simulink model "Test_JI_dot_dot"  (R2015b)
settings: Solver=ode4  StartTime=0.0  StopTime=10  FixedStep=0.01  RelTol=1e-3
values from neighbouring files (symbols this model uses):
  D = [30,30,20,20,20,20,20,20]    [Set_Parameter.m]    (also in Set_Parameter_Single.m; Set_Parameter_line_circle.m; Set_Parameter_line_circle_DC_model_no_vision_controller.m; Set_Parameter_line_circle_no_vision_controller.m = [40,40,40,30,20,30,20,20])
  P = [60,60,50,50,30,30,20,20]    [Set_Parameter.m]    (also in Set_Parameter_Single.m; Set_Parameter_line_circle.m; Set_Parameter_line_circle_DC_model_no_vision_controller.m = [120,120,100,100,60,60,40,40]; Set_Parameter_line_circle_no_vision_controller.m = [350,100,300,150,50,100,20,20])
settings Model: Creator=User  LastModifiedBy=User

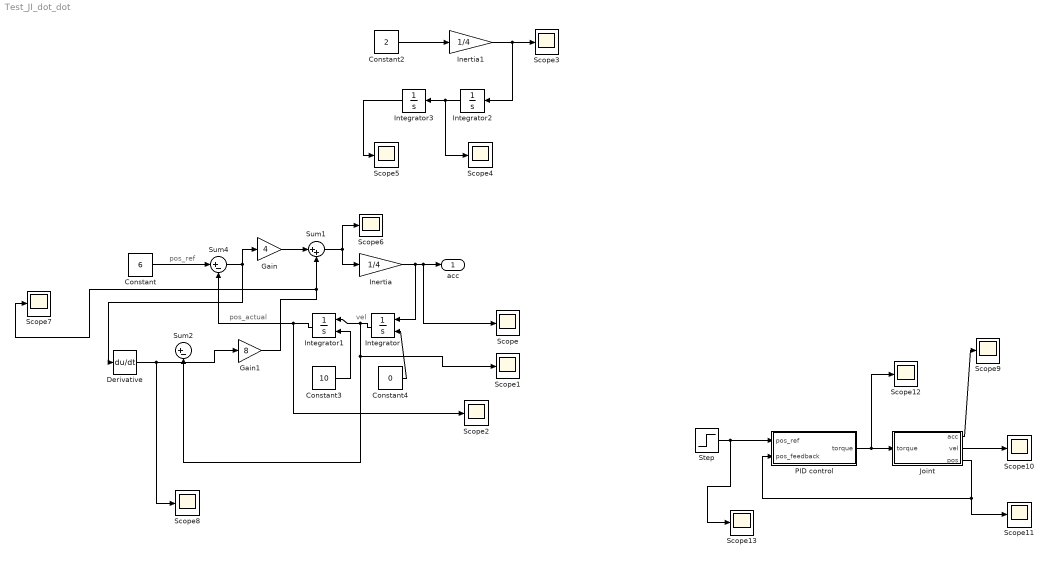
== system Test_JI_dot_dot ==
  note: pos_ref
  note: pos_actual
  note: vel
  Constant : Constant  Value=6
  Constant2 : Constant  Value=2
  Constant3 : Constant  Value=10
  Constant4 : Constant  Value=0
  Derivative : Derivative
  Gain : Gain  Gain=4
  Gain1 : Gain  Gain=8
  Inertia : Gain  Gain=1/4
  Inertia1 : Gain  Gain=1/4
  Integrator : Integrator  InitialConditionSource=external
  Integrator1 : Integrator  InitialConditionSource=external
  Integrator2 : Integrator
  Integrator3 : Integrator
  Joint : Subsystem
  PID control : Subsystem
  Scope{,1..13} (14 alike) : Scope
  Step : Step  After=6  SampleTime=0
  Sum1 : Sum  Inputs=|++
  Sum2 : Sum  Inputs=|+-
  Sum4 : Sum  Inputs=|+-
  acc : Outport
  wires:
  Inertia/1 -> Integrator/1, Scope/1, acc/1
  Integrator/1 -> Sum2/2, Scope1/1, Integrator1/1
  Integrator1/1 -> Scope2/1, Sum4/2
  Constant/1 -> Sum4/1
  Sum4/1 -> Derivative/1, Gain/1
  Gain/1 -> Sum1/1
  Sum1/1 -> Inertia/1, Scope6/1
  Constant2/1 -> Inertia1/1
  Inertia1/1 -> Integrator2/1, Scope3/1
  Integrator2/1 -> Integrator3/1, Scope4/1
  Integrator3/1 -> Scope5/1
  Constant3/1 -> Integrator1/2
  Constant4/1 -> Integrator/2
  Gain1/1 -> Scope7/1, Sum1/2
  Derivative/1 -> Gain1/1, Scope8/1
  Step/1 -> Scope13/1, PID control/1("pos_ref ")
  PID control/1(torque) -> Scope12/1, Joint/1(torque)
  Joint/3(pos) -> Scope11/1, PID control/2(pos_feedback)
  Joint/1(acc) -> Scope9/1
  Joint/2(vel) -> Scope10/1

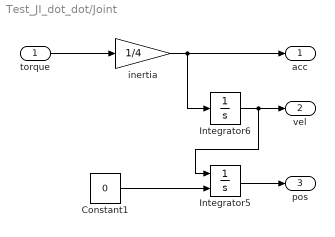
== system Test_JI_dot_dot/Joint ==
  torque : Inport
  Constant1 : Constant  Value=0
  Integrator5 : Integrator  InitialConditionSource=external
  Integrator6 : Integrator
  inertia : Gain  Gain=1/4
  acc : Outport
  vel : Outport  Port=2
  pos : Outport  Port=3
  wires:
  inertia/1 -> Integrator6/1, acc/1
  torque/1 -> inertia/1
  Constant1/1 -> Integrator5/2
  Integrator6/1 -> vel/1, Integrator5/1
  Integrator5/1 -> pos/1

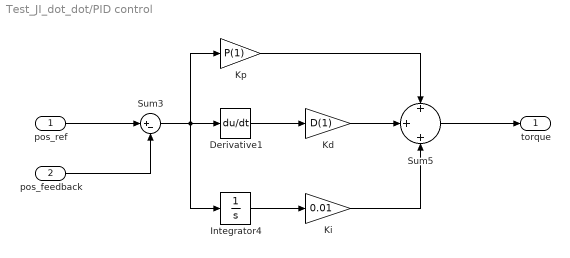
== system Test_JI_dot_dot/PID control ==
  "pos_ref " : Inport
  pos_feedback : Inport  Port=2
  Derivative1 : Derivative
  Integrator4 : Integrator
  Kd : Gain  Gain=D(1)
  Ki : Gain  Gain=0.01
  Kp : Gain  Gain=P(1)
  Sum3 : Sum  Inputs=|+-
  Sum5 : Sum  Inputs=+|+|+
  torque : Outport
  wires:
  Sum5/1 -> torque/1
  Integrator4/1 -> Ki/1
  Ki/1 -> Sum5/3
  Kp/1 -> Sum5/1
  "pos_ref "/1 -> Sum3/1
  Sum3/1 -> Integrator4/1, Derivative1/1, Kp/1
  Kd/1 -> Sum5/2
  Derivative1/1 -> Kd/1
  pos_feedback/1 -> Sum3/2
